simulink model "Lab1PartA3"  (R2016a)
settings: Solver=VariableStepAuto  StartTime=0.0  StopTime=20.0  RelTol=1e-3
settings Model: Creator=pzastawn  LastModifiedBy=pzastawn

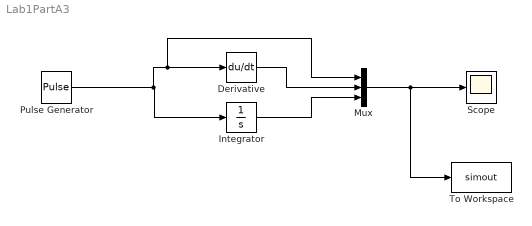
== system Lab1PartA3 ==
  Derivative : Derivative
  Integrator : Integrator
  Mux : Mux  Inputs=3
  Pulse Generator : DiscretePulseGenerator  PulseType=Time based  Period=5  PulseWidth=50
  Scope : Scope
  To Workspace : ToWorkspace  VariableName=simout  SaveFormat=Timeseries  SampleTime=-1
  wires:
  Pulse Generator/1 -> Mux/1, Derivative/1, Integrator/1
  Mux/1 -> To Workspace/1, Scope/1
  Derivative/1 -> Mux/2
  Integrator/1 -> Mux/3
